simulink library "relay_tripOutMng_lib"  (Simulink 8.1)
settings: Solver=ode45  StartTime=0.0  StopTime=10.0  RelTol=1e-3
libraries: simulink x3, simulink_extras x2
settings Model: Creator=RE25624  LastModifiedBy=re25624

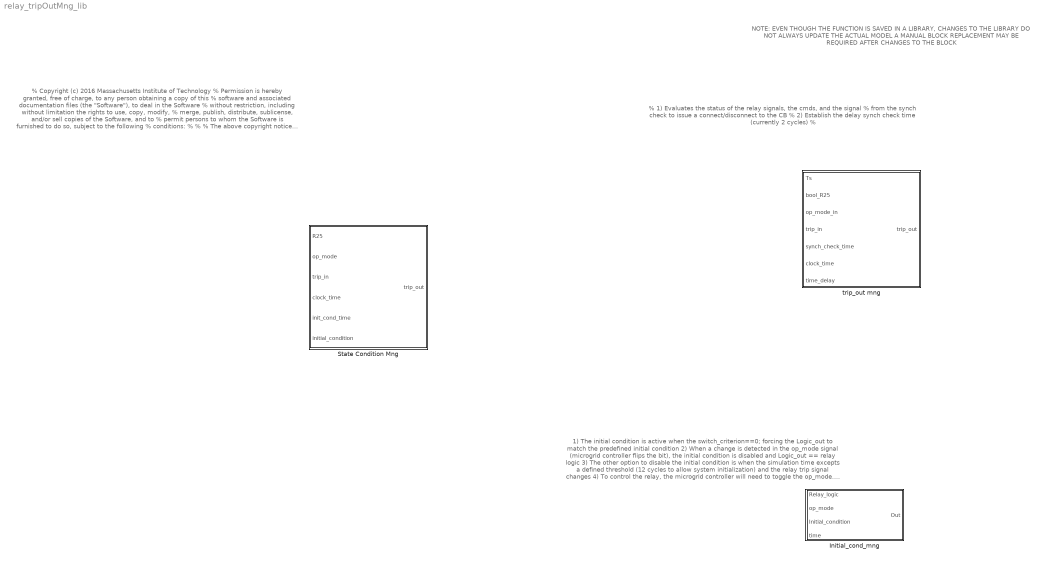
== system relay_tripOutMng_lib ==
  note: NOTE:  EVEN THOUGH THE FUNCTION IS SAVED IN A LIBRARY, CHANGES TO THE LIBRARY DO NOT ALWAYS UPDATE THE ACTUAL MODEL
      |
      | A MANUAL BLOCK REPLACEMENT MAY BE REQUIRED AFTER CHANGES TO THE BLOCK
  note: % 1) Evaluates the status of the relay signals, the cmds, and the signal
      | % from the synch check to issue a connect/disconnect to the CB
      | % 2) Establish the delay synch check time (currently 2 cycles)
      | %
  note: % Copyright (c) 2016 Massachusetts Institute of Technology
      | % Permission is hereby granted, free of charge, to any person obtaining a copy of this
      | % software and associated documentation files (the "Software"), to deal in the Software
      | % without restriction, including without limitation the rights to use, copy, modify,
      | % merge, publish, distribute, sublicense, and/or sell copies of the Software, and to
      | % permit persons to whom the Software is furnished to do so, subject to the following
      | % conditions:
      | %
      | %
      | % The above copyright notice and this permission notice shall be included in
      | % all copies or substantial portions of the Software.
      | %
      | % THE SOFTWARE IS PROVIDED "AS IS", WITHOUT WARRANTY OF ANY KIND, EXPRESS OR IMPLIED,
      | % INCLUDING BUT NOT LIMITED TO THE WARRANTIES OF MERCHANTABILITY, FITNESS FOR A
      | % PARTICULAR PURPOSE AND NONINFRINGEMENT. IN NO EVENT SHALL THE AUTHORS OR COPYRIGHT
      | % HOLDERS BE LIABLE FOR ANY CLAIM, DAMAGES OR OTHER LIABILITY, WHETHER IN AN ACTION
      | % OF CONTRACT, TORT OR OTHERWISE, ARISING FROM, OUT OF OR IN CONNECTION WITH THE
      | % SOFTWARE OR THE USE OR OTHER DEALINGS IN THE SOFTWARE.
      | %
      | %
      | %%
  note: 1) The initial condition is active when the switch_criterion==0; forcing the Logic_out to match the predefined initial condition
      | 2) When a change is detected in the op_mode signal (microgrid controller flips the bit), the initial condition is disabled
      | and Logic_out == relay logic
      | 3) The other option to disable the initial condition is when the simulation time excepts a defined threshold (12 cycles to allow system initialization) and the relay trip signal changes
      | 4) To control the relay, the microgrid controller will need to toggle the op_mode. Say 0 -> 1 -> 0
  Initial_cond_mng : Subsystem  mask(Initial Condition Management){initCond_hold_time=0.2}
      mask prompts: initCond_hold_time "Initial Condition Threshold Time [Secs]"
      mask help: Initial Condition Threshold Time [Secs]: Time in second the relay will hold its defined initial condition. The initial condition may be used to allow the system to reach initial steady-state
  State Condition Mng : Subsystem
  trip_out mng : MATLAB Function  TreatAsAtomicUnit=on

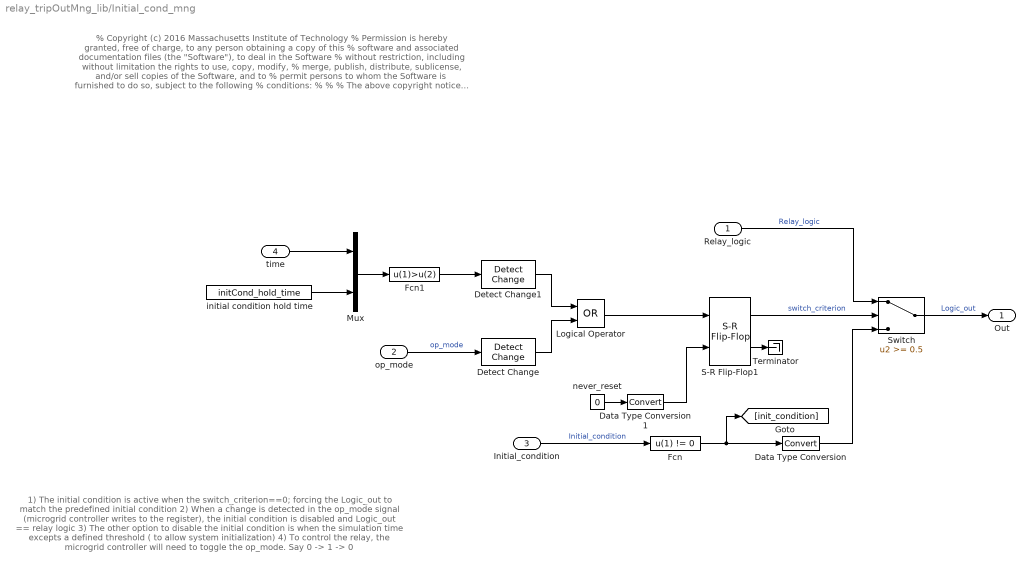
== system relay_tripOutMng_lib/Initial_cond_mng ==
  note: % Copyright (c) 2016 Massachusetts Institute of Technology
      | % Permission is hereby granted, free of charge, to any person obtaining a copy of this
      | % software and associated documentation files (the "Software"), to deal in the Software
      | % without restriction, including without limitation the rights to use, copy, modify,
      | % merge, publish, distribute, sublicense, and/or sell copies of the Software, and to
      | % permit persons to whom the Software is furnished to do so, subject to the following
      | % conditions:
      | %
      | %
      | % The above copyright notice and this permission notice shall be included in
      | % all copies or substantial portions of the Software.
      | %
      | % THE SOFTWARE IS PROVIDED "AS IS", WITHOUT WARRANTY OF ANY KIND, EXPRESS OR IMPLIED,
      | % INCLUDING BUT NOT LIMITED TO THE WARRANTIES OF MERCHANTABILITY, FITNESS FOR A
      | % PARTICULAR PURPOSE AND NONINFRINGEMENT. IN NO EVENT SHALL THE AUTHORS OR COPYRIGHT
      | % HOLDERS BE LIABLE FOR ANY CLAIM, DAMAGES OR OTHER LIABILITY, WHETHER IN AN ACTION
      | % OF CONTRACT, TORT OR OTHERWISE, ARISING FROM, OUT OF OR IN CONNECTION WITH THE
      | % SOFTWARE OR THE USE OR OTHER DEALINGS IN THE SOFTWARE.
      | %
      | %
      | %%
  note: 1) The initial condition is active when the switch_criterion==0; forcing the Logic_out to match the predefined initial condition
      | 2) When a change is detected in the op_mode signal (microgrid controller writes to the register), the initial condition is disabled and Logic_out == relay logic
      | 3) The other option to disable the initial condition is when the simulation time excepts a defined threshold ( to allow system initialization)
      | 4) To control the relay, the microgrid controller will need to toggle the op_mode. Say 0 -> 1 -> 0
  Relay_logic : Inport
  op_mode : Inport  Port=2
  Initial_condition : Inport  Port=3
  time : Inport  Port=4
  Data Type Conversion : DataTypeConversion
  Data Type Conversion1 : DataTypeConversion
  Detect Change : simulink/Logic and Bit Operations/Detect Change  vinit=0  InputProcessing=Inherited  OutDataTypeStr=boolean
  Detect Change1 : simulink/Logic and Bit Operations/Detect Change  vinit=0  InputProcessing=Inherited  OutDataTypeStr=boolean
  Fcn : Fcn  Expr=u(1) != 0
  Fcn1 : Fcn  Expr=u(1)>u(2)
  Logical Operator : Logic  Operator=OR  AllPortsSameDT=off  OutDataTypeStr=boolean
  Mux : Mux  Inputs=2
  S-R Flip-Flop1 : simulink_extras/Flip Flops/S-R Flip-Flop  initial_condition=0
  Switch : Switch  Threshold=0.5
  Terminator : Terminator
  initial condition hold time : Constant  Value=initCond_hold_time
  never_reset : Constant  Value=0
  Out : Outport
  wires:
  initial condition hold time/1 -> Mux/2
  Logical Operator/1 -> S-R Flip-Flop1/1
  Detect Change/1 -> Logical Operator/2
  Detect Change1/1 -> Logical Operator/1
  Fcn1/1 -> Detect Change1/1
  time/1 -> Mux/1
  Mux/1 -> Fcn1/1
  Relay_logic/1 -> Switch/1  "Relay_logic"
  Data Type Conversion/1 -> Switch/3
  Initial_condition/1 -> Fcn/1  "Initial_condition"
  Fcn/1 -> Data Type Conversion/1, [init_condition]
  S-R Flip-Flop1/1 -> Switch/2  "switch_criterion"
  S-R Flip-Flop1/2 -> Terminator/1
  Switch/1 -> Out/1  "Logic_out"
  Data Type Conversion1/1 -> S-R Flip-Flop1/2
  op_mode/1 -> Detect Change/1  "op_mode"
  never_reset/1 -> Data Type Conversion1/1

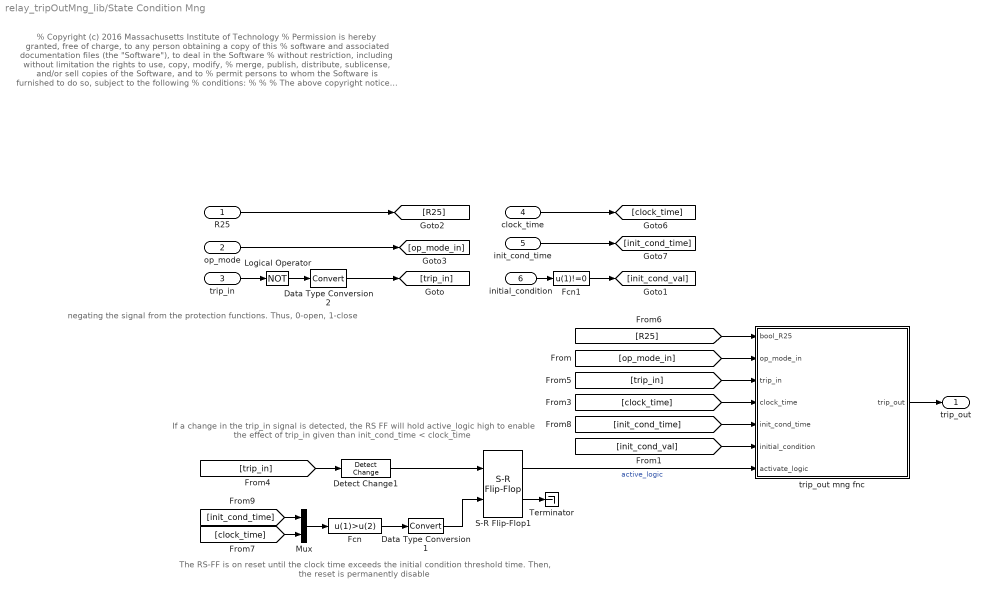
== system relay_tripOutMng_lib/State Condition Mng ==
  note: negating the signal from the protection functions.
      | Thus, 0-open, 1-close
  note: % Copyright (c) 2016 Massachusetts Institute of Technology
      | % Permission is hereby granted, free of charge, to any person obtaining a copy of this
      | % software and associated documentation files (the "Software"), to deal in the Software
      | % without restriction, including without limitation the rights to use, copy, modify,
      | % merge, publish, distribute, sublicense, and/or sell copies of the Software, and to
      | % permit persons to whom the Software is furnished to do so, subject to the following
      | % conditions:
      | %
      | %
      | % The above copyright notice and this permission notice shall be included in
      | % all copies or substantial portions of the Software.
      | %
      | % THE SOFTWARE IS PROVIDED "AS IS", WITHOUT WARRANTY OF ANY KIND, EXPRESS OR IMPLIED,
      | % INCLUDING BUT NOT LIMITED TO THE WARRANTIES OF MERCHANTABILITY, FITNESS FOR A
      | % PARTICULAR PURPOSE AND NONINFRINGEMENT. IN NO EVENT SHALL THE AUTHORS OR COPYRIGHT
      | % HOLDERS BE LIABLE FOR ANY CLAIM, DAMAGES OR OTHER LIABILITY, WHETHER IN AN ACTION
      | % OF CONTRACT, TORT OR OTHERWISE, ARISING FROM, OUT OF OR IN CONNECTION WITH THE
      | % SOFTWARE OR THE USE OR OTHER DEALINGS IN THE SOFTWARE.
      | %
      | %
      | %%
  note: The RS-FF is on reset until the clock time exceeds the initial condition threshold time.
      | Then, the reset is permanently disable
  note: If a change in the trip_in signal is detected, the RS FF will hold active_logic high
      |  to enable the effect of trip_in given than init_cond_time < clock_time
  R25 : Inport
  op_mode : Inport  Port=2
  trip_in : Inport  Port=3
  clock_time : Inport  Port=4
  init_cond_time : Inport  Port=5
  initial_condition : Inport  Port=6
  Data Type Conversion1 : DataTypeConversion
  Data Type Conversion2 : DataTypeConversion
  Detect Change1 : simulink/Logic and Bit Operations/Detect Change  vinit=0  InputProcessing=Inherited  OutDataTypeStr=boolean
  Fcn : Fcn  Expr=u(1)>u(2)
  Fcn1 : Fcn  Expr=u(1)!=0
  Logical Operator : Logic  Operator=NOT  AllPortsSameDT=off  OutDataTypeStr=boolean
  Mux : Mux  Inputs=2
  S-R Flip-Flop1 : simulink_extras/Flip Flops/S-R Flip-Flop  initial_condition=0
  Terminator : Terminator
  trip_out mng fnc : MATLAB Function  TreatAsAtomicUnit=on
  trip_out : Outport
  wires:
  Data Type Conversion2/1 -> [trip_in]
  Logical Operator/1 -> Data Type Conversion2/1
  trip_in/1 -> Logical Operator/1
  Fcn1/1 -> [init_cond_val]
  [init_cond_val] -> trip_out mng fnc/6(initial_condition)
  initial_condition/1 -> Fcn1/1
  S-R Flip-Flop1/1 -> trip_out mng fnc/7(activate_logic)  "active_logic"
  [init_cond_time] -> Mux/1
  [clock_time] -> Mux/2
  [init_cond_time] -> trip_out mng fnc/5(init_cond_time)
  Fcn/1 -> Data Type Conversion1/1
  Mux/1 -> Fcn/1
  Data Type Conversion1/1 -> S-R Flip-Flop1/2
  [trip_in] -> trip_out mng fnc/3(trip_in)
  S-R Flip-Flop1/2 -> Terminator/1
  Detect Change1/1 -> S-R Flip-Flop1/1
  [trip_in] -> Detect Change1/1
  [clock_time] -> trip_out mng fnc/4(clock_time)
  R25/1 -> [R25]
  [R25] -> trip_out mng fnc/1(bool_R25)
  init_cond_time/1 -> [init_cond_time]
  [op_mode_in] -> trip_out mng fnc/2(op_mode_in)
  clock_time/1 -> [clock_time]
  op_mode/1 -> [op_mode_in]
  trip_out mng fnc/1(trip_out) -> trip_out/1

== matlab function State Condition Mng/trip_out mng fnc ==
  data: bool_R25 input double; op_mode_in input double; trip_out output double; trip_in input double; clock_time input double; init_cond_time input double; initial_condition input double; activate_logic input double
% Copyright (c) 2016 Massachusetts Institute of Technology
% Permission is hereby granted, free of charge, to any person obtaining a copy of this
% software and associated documentation files (the "Software"), to deal in the Software
% without restriction, including without limitation the rights to use, copy, modify,
% merge, publish, distribute, sublicense, and/or sell copies of the Software, and to
% permit persons to whom the Software is furnished to do so, subject to the following
% conditions:
%
%
% The above copyright notice and this permission notice shall be included in
% all copies or substantial portions of the Software.
%
% THE SOFTWARE IS PROVIDED "AS IS", WITHOUT WARRANTY OF ANY KIND, EXPRESS OR IMPLIED,
% INCLUDING BUT NOT LIMITED TO THE WARRANTIES OF MERCHANTABILITY, FITNESS FOR A
% PARTICULAR PURPOSE AND NONINFRINGEMENT. IN NO EVENT SHALL THE AUTHORS OR COPYRIGHT
% HOLDERS BE LIABLE FOR ANY CLAIM, DAMAGES OR OTHER LIABILITY, WHETHER IN AN ACTION
% OF CONTRACT, TORT OR OTHERWISE, ARISING FROM, OUT OF OR IN CONNECTION WITH THE
% SOFTWARE OR THE USE OR OTHER DEALINGS IN THE SOFTWARE.
%
%
%%

function trip_out = opModeChk(bool_R25, op_mode_in, trip_in, clock_time, init_cond_time, initial_condition, activate_logic)
%#codegen

% PARAMETERS:
% bool_R25 - synch-check: indication of CB terminal being in synch as per the specified relay settings.
% op_mode_in: signal from MGC on how to operate the relay/CB
% op_mode_in = [0-close/logic, 1-close/no-logic, 2-open]
% trip_in: signal from protection elements depending on system conditions
% trip_in = (0-trip cb, 1-close cb)
% clock_time: simulation clock time
% init_cond_time[s]: predefined time to hold the initial condition
% initial_condition: relay setting indicating the initial state of the CB
% initial_condition = [0-open, 1-close]
% activate_logic: bool signal indicating to switch from initial condition
% to the actual logic (0-init_cond, 1-logic)
% trip_out: 0-open the cb, 1-close the cb

% the trip_out signal will equal the initial_condition until the simulation
% clock time exceeds the initial condition time requierements and
% active_logic is true
trip_out = initial_condition;

if (clock_time > init_cond_time) && activate_logic
    
    if op_mode_in == 0
        % if conditions to apply the trip_in signal are met, and the
        % operation mode dictated by the MGC is 0-logic, and the terminals
        % of the CB are in synch (under specified conditions). Then, CB
        % will receive a close signal while allowing the protection
        % functions to operate and open the CB if necessary
        trip_out = trip_in * bool_R25;
    elseif op_mode_in == 1
        % if conditions to apply the trip_in signal are met, and the
        % operation mode dictated by the MGC is 0-close, and the terminals
        % of the CB are in synch (under specified conditions).  Then, CB
        % will receive a close signal while disabling the protection
        % functions. The CB will remain closed as long as the synch-check
        % verifies synchronism between terminals
        trip_out = 1 * bool_R25;
    elseif op_mode_in == 2
        % if the operation mode dictated by the MGC is 2-open, the CB will
        % receive an open command
        trip_out = 0;
    end
end

== matlab function trip_out mng ==
  data: Ts input double; bool_R25 input double; op_mode_in input double; trip_out output double; trip_in input double; synch_check_time input double; clock_time input double; time_delay input double
% Copyright (c) 2016 Massachusetts Institute of Technology
% Permission is hereby granted, free of charge, to any person obtaining a copy of this 
% software and associated documentation files (the "Software"), to deal in the Software
% without restriction, including without limitation the rights to use, copy, modify, 
% merge, publish, distribute, sublicense, and/or sell copies of the Software, and to 
% permit persons to whom the Software is furnished to do so, subject to the following 
% conditions:
% 
% 
% The above copyright notice and this permission notice shall be included in 
% all copies or substantial portions of the Software.
% 
% THE SOFTWARE IS PROVIDED "AS IS", WITHOUT WARRANTY OF ANY KIND, EXPRESS OR IMPLIED, 
% INCLUDING BUT NOT LIMITED TO THE WARRANTIES OF MERCHANTABILITY, FITNESS FOR A 
% PARTICULAR PURPOSE AND NONINFRINGEMENT. IN NO EVENT SHALL THE AUTHORS OR COPYRIGHT 
% HOLDERS BE LIABLE FOR ANY CLAIM, DAMAGES OR OTHER LIABILITY, WHETHER IN AN ACTION 
% OF CONTRACT, TORT OR OTHERWISE, ARISING FROM, OUT OF OR IN CONNECTION WITH THE 
% SOFTWARE OR THE USE OR OTHER DEALINGS IN THE SOFTWARE.
%
%
%%

% 1) Evaluates the status of the relay signals, the cmds, and the signal
% from the synch check to issue a connect/disconnect to the CB
% 2) Establish the delay synch check time (currently 2 cycles)
%

function trip_out = opModeChk(Ts, bool_R25, op_mode_in, trip_in, synch_check_time, clock_time, time_delay)
%#codegen

persistent n25 prev_mode prev_trip_in
if isempty(prev_mode)
    n25 = 0; % time counter
    prev_mode = 0; % initially operating on logic
    prev_trip_in = 1; % initially close
end

trip_out = trip_in * bool_R25;

% the R25 logic will be active if the breaker has been opened, and a
% forced-to-close command is applied
if (prev_mode==2 || prev_trip_in==0) && (op_mode_in==1 || op_mode_in==0) && trip_in==1
    
    % time accumulation
    n25 = n25 * bool_R25;
    n25 = n25 + bool_R25 * Ts;
    if n25 > synch_check_time
        trip_out = 1;
        % reset history values
        prev_mode = op_mode_in;
        prev_trip_in = trip_in;
    else
        prev_mode = 2;
        prev_trip_in = 0;
        trip_out = 0;
    end
    
elseif op_mode_in==2
    prev_mode = 2;
    prev_trip_in = 0;
    trip_out = 0;
    n25 = 0;
else
    n25 = 0;
end


% time delay [sec] to activate logic. Forces the trip_out signal
% to 1 (close) until the simulation clock exceeds the threshold
if clock_time < time_delay
    trip_out = 1;
end
